simulink model "ScriptDemo"  (R2022b)
settings: configuration reference "TmVcThermal_Configuration_sub" (kept outside this file)
undefined symbols (not defined in the file or in its folder): aaaa, bbbb, cTmComprCtrl_D_u8HvacFlowTable_db, cTmComprCtrl_D_u8HvacFlowTable_sw, cTmComprCtrl_n_i16ChillCmpIMax, cTmComprCtrl_n_i16ChillCmpIMin, cTmComprCtrl_n_i16ChillCmpIMin666, cTmComprCtrl_n_i16ChillCmpPMax, cTmComprCtrl_n_i16ChillCmpPMin, cTmComprCtrl_n_i16CmpChillCoolRpmKiMax, cTmComprCtrl_n_i16CmpChillCoolRpmKiMin, cTmComprCtrl_n_i16CmpChillCoolRpmKpMax, cTmComprCtrl_n_i16CmpChillCoolRpmKpMin, cTmComprCtrl_n_i16CmpCoolRpmKiMax, cTmComprCtrl_n_i16CmpCoolRpmKiMin, cTmComprCtrl_n_i16CmpCoolRpmKpMax, cTmComprCtrl_n_i16CmpCoolRpmKpMin, cTmComprCtrl_n_i16SM4CmpHeatKiMax, cTmComprCtrl_n_i16SM4CmpHeatKiMin, cTmComprCtrl_n_i16SM4CmpHeatKpMax, cTmComprCtrl_n_i16SM4CmpHeatKpMin, cTmComprCtrl_n_i16SM5CmpHeatKiMax, cTmComprCtrl_n_i16SM5CmpHeatKiMin, cTmComprCtrl_n_i16SM5CmpHeatKpMax, cTmComprCtrl_n_i16SM5CmpHeatKpMin, cTmComprCtrl_n_i16SM6CmpHeatKiMax, cTmComprCtrl_n_i16SM6CmpHeatKiMin, cTmComprCtrl_n_i16SM6CmpHeatKpMax, cTmComprCtrl_n_i16SM6CmpHeatKpMin, cTmComprCtrl_n_u16CmpMaxSpdFanFltLimt, cTmComprCtrl_n_u16CmpMaxSpdLoSidePFltLimt, cTmComprCtrl_n_u16CmpMaxSpdSensorFltLimt, cTmComprCtrl_n_u16CompMinRpm, cTmComprCtrl_n_u16CompRpmIncThres, cTmComprCtrl_t_u16BattCooltFFPeriod, cTmComprCtrl_t_u16BattCooltPIPeriod, cTmComprCtrl_t_u16CmpCoolFFPeriod, cTmComprCtrl_t_u16CmpCoolPIPeriod, cTmComprCtrl_t_u16CoolCmpChillFFPeriod, cTmComprCtrl_t_u16CoolCmpChillPIPeriod, cTmComprCtrl_t_u16SM4CmpHeatFFPeriod, cTmComprCtrl_t_u16SM4CmpHeatPIPeriod, cTmComprCtrl_t_u16SM5CmpHeatFFPeriod, cTmComprCtrl_t_u16SM5CmpHeatPIPeriod, cTmComprCtrl_t_u16SM6CmpHeatFFPeriod, cTmComprCtrl_t_u16SM6CmpHeatPIPeriod, cTmComprCtrl_Te_EvapClearInteg, cTmComprCtrl_Te_i16HpReqTempSaturoffset, cTmComprCtrl_Te_i16SatLpReplaceDiff, cTmComprCtrl_Te_i16SM3BatDiffStartEvapDecOffset, cTmComprCtrl_Te_i16SM3EvapLo, cTmComprCtrl_Te_i16SM3TBatDiffEntEvapDecOffset, cTmComprCtrl_Te_i16SM3TBatDiffEntEvapDecOffsetQuit, cTmComprCtrl_Te_s32ErrCmpChillPIContinueCoolH, cTmComprCtrl_Te_s32ErrCmpChillPIContinueCoolL, cTmComprCtrl_Te_s32ErrCmpPIContinueChillH, cTmComprCtrl_Te_s32ErrCmpPIContinueChillL, cTmComprCtrl_Te_s32ErrCmpPIContinueCoolH, cTmComprCtrl_Te_s32ErrCmpPIContinueCoolL, cTmComprCtrl_Te_s32ErrCmpPIContinueHeatH ... (+398)
libraries: simulink x846, PCMULib x711, simulink_need_slupdate x4
(part 1 of 49)
settings Model: PacingRate=56  Creator=blue.ge  LastModifiedBy=blue.ge
settings ConfigSetRef: SourceName=TmVcThermal_Configuration_sub  SourceLocation=Base Workspace

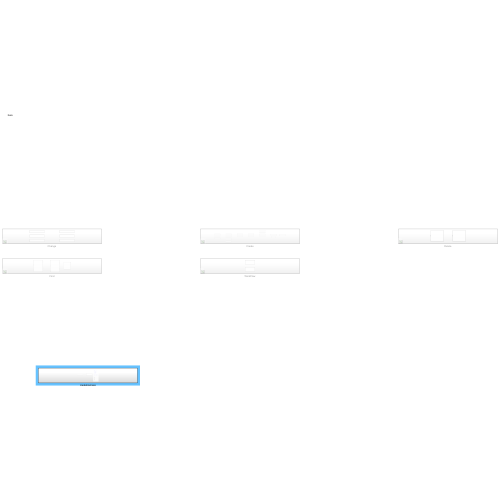
[thumbnail: Simulink's stored preview of the top-level diagram]
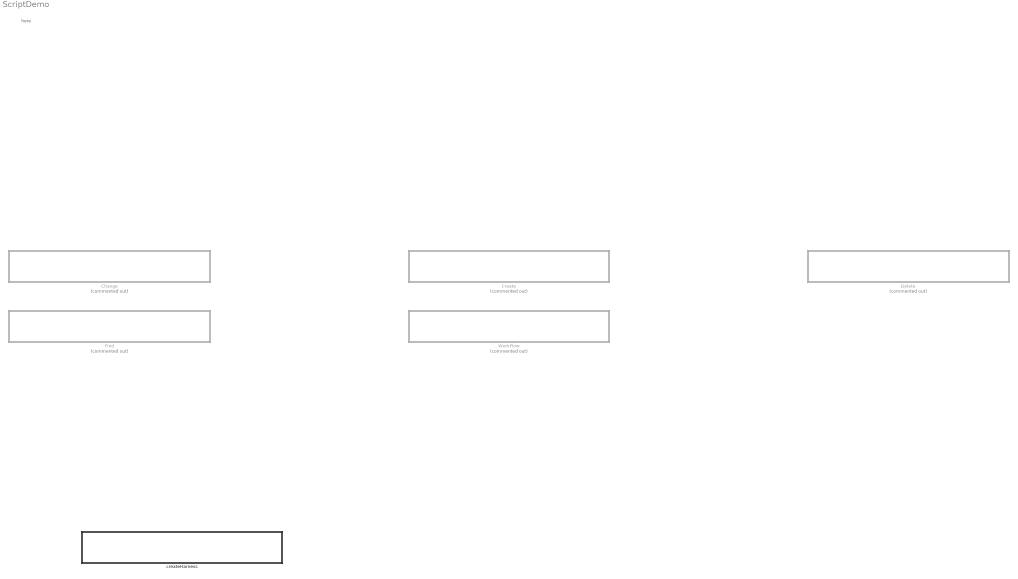
== system ScriptDemo ==
  note: here
  Change : Subsystem  Commented=on
  Create : Subsystem  Commented=on
  Delete : Subsystem  Commented=on
  Find : Subsystem  Commented=on
  WorkFlow : Subsystem  Commented=on
  createHarness : Subsystem

== system ScriptDemo/Change ==
  changeModPortName : Subsystem
  changeModPortType : Subsystem
  changeModSize : Subsystem
  changeModSizeGcs : Subsystem
  changePortBlockPosAll : Subsystem
  changeSigType : Subsystem

== system ScriptDemo/Create ==
  Model : Subsystem
  creatIFIn : Subsystem
  creatIFOut : Subsystem
  creatTmBase : Subsystem
  creatTmBaseArch : Subsystem
  creatTmIn : Subsystem
  creatTmOut : Subsystem
  createBus : Subsystem
  createDebug : Subsystem
  createGotoBasedPorts : Subsystem
  createGotoUseless : Subsystem
  createHarness : Subsystem
  createMerge : Subsystem
  createPorts : Subsystem
  createSigOnLine : Subsystem
  createStoreMem : Subsystem
  createSubMod : Subsystem
  createSubmodInfo : Subsystem
  createSwitchCase : Subsystem

== system ScriptDemo/Delete ==
  delUselessLine : Subsystem
  delUselessPort : Subsystem

== system ScriptDemo/Find ==
  findModBkConnected : Subsystem
  findModBkSpecific : Subsystem
  findNameMdOut : Subsystem

== system ScriptDemo/WorkFlow ==
  Step1_CreateSoftwareReq : Subsystem
  Step1_CreateSubModel : Subsystem

== system ScriptDemo/createHarness ==
  note: % 运行此脚本的时候，需要确保模型仿真通过, 可临时屏蔽其它案例或者将此模型复制到新的空白模型中
      |
      | createHarness(gcb, ...
      | 'lastStep' , 'Initialize' , ... % Initialize
      | 'mask' ,false, ...
      | 'lev1' ,{ 'NHP' , 'HP' }, ...
      | 'lev2' ,{ ...
      | { 'NoLimit' , 'Limit' }, ...
      | { 'NoLimit' , 'Limit' , 'Limit2' , 'Limit3' }, ...
      | }, ...
      | 'inName' ,{ ...
      | {
      | 'sTmIn_D_u8HeatPump' , ...
      | 'sTmDiag_D_u8HiSidePNHPFltSt' , ...
      | }, ...
      | {
      | 'sTmIn_D_u8HeatPump' , ...
      | 'sTmDiag_D_u8HiSidePFltSt' , ...
      | 'sTmDiag_D_u8OutrCondOutTFltSt' , ...
      | 'sTmDiag_D_u8CmprDischrgTFltSt' , ...
      | }, ...
      | }, ...
      | 'rstName' ,{ ...
      | {
      | 'rTmComprCtrl_n_u16CompMaxRpmSensFlt' ...
      | 'xTmComprCtrl_B_CmpSensorFltLimtFlag' ...
      | }, ...
      | {
      | 'rTmComprCtrl_n_u16CompMaxRpmSensFlt' ...
      | 'xTmComprCtrl_B_CmpSensorFltLimtFlag' ...
      | }, ...
      | }, ...
      | 'inValue' ,{ ...
      | { ...
      | {1 0 }, ...
      | {1 [1 2 3] }, ...
      | }, ...
      | { ...
      | {2 0 0 0 }, ...
      | {2 1 0 0 }, ...
      | {2 0 1 0 }, ...
      | {2 0 0 1 }, ...
      | }, ...
      | }, ...
      | 'rstValue' ,{ ...
      | { ...
      | {8000 false}, ...
      | {3000 true}, ...
      | }, ...
      | { ...
      | {8000 false}, ...
      | {3000 true}, ...
      | {3000 true}, ...
      | {3000 true}, ...
      | }, ...
      | } ...
      | )
  After : Subsystem
  Before : Subsystem  Commented=on
  Blue : Subsystem  Commented=on
  ID31659_OffCodeState : Subsystem

== system ScriptDemo/Change/changeModPortName ==
  After : Subsystem
  Before : Subsystem

== system ScriptDemo/Change/changeModPortType ==
  After : Subsystem
  Before : Subsystem

== system ScriptDemo/Change/changeModSize ==
  After : Subsystem
  Before : Subsystem

== system ScriptDemo/Change/changeModSizeGcs ==
  Before : Subsystem
  Before1 : Subsystem

== system ScriptDemo/Change/changePortBlockPosAll ==
  After1 : Subsystem
  Before : Subsystem

== system ScriptDemo/Change/changeSigType ==
  Before : Subsystem
  Before1 : Subsystem

== system ScriptDemo/Create/Model ==
  createModGoto : Subsystem
  createModGotoAll : Subsystem
  createModGroundTerm : Subsystem
  createModPorts : Subsystem
  createModSig : Subsystem
  createMode : Subsystem

== system ScriptDemo/Create/creatIFIn ==
  After : Subsystem
  Before : Subsystem

== system ScriptDemo/Create/creatIFOut ==
  After : Subsystem
  Before : Subsystem

== system ScriptDemo/Create/creatTmBase ==
  After : Subsystem
  Before : Subsystem

== system ScriptDemo/Create/creatTmBaseArch ==
  After : Subsystem
  Before : Subsystem

== system ScriptDemo/Create/creatTmIn ==
  After : Subsystem
  Before : Subsystem

== system ScriptDemo/Create/creatTmOut ==
  Before : Subsystem
  TmBase2Out : Subsystem
  wires:
  [sTmComprCtrl_n_u16CompRpmReq] -> TmBase2Out/1(sTmComprCtrl_n_u16CompRpmReq)
  [yTmComprCtrl_B_CompOnReq] -> TmBase2Out/2(yTmComprCtrl_B_CompOnReq)
  [sTmEnergyMgr_Pw_s32AcCmprPwrLim] -> TmBase2Out/3(sTmEnergyMgr_Pw_s32AcCmprPwrLim)
  [sTmRefriVlvCtrl_X_s32EEXVPosReq] -> TmBase2Out/4(sTmRefriVlvCtrl_X_s32EEXVPosReq)
  [yTmRefriVlvCtrl_B_EexvCalibReq] -> TmBase2Out/5(yTmRefriVlvCtrl_B_EexvCalibReq)
  [yTmRefriVlvCtrl_B_HpcEexvMovEnable] -> TmBase2Out/6(yTmRefriVlvCtrl_B_HpcEexvMovEnable)
  [sTmRefriVlvCtrl_X_s32BEXVPosReq] -> TmBase2Out/7(sTmRefriVlvCtrl_X_s32BEXVPosReq)
  [yTmRefriVlvCtrl_B_BexvCalibReq] -> TmBase2Out/8(yTmRefriVlvCtrl_B_BexvCalibReq)
  [yTmRefriVlvCtrl_B_HpcBexvMovEnable] -> TmBase2Out/9(yTmRefriVlvCtrl_B_HpcBexvMovEnable)
  [sTmRefriVlvCtrl_X_s32CEXVPosReq] -> TmBase2Out/10(sTmRefriVlvCtrl_X_s32CEXVPosReq)
  [yTmRefriVlvCtrl_B_CexvCalibReq] -> TmBase2Out/11(yTmRefriVlvCtrl_B_CexvCalibReq)
  [yTmRefriVlvCtrl_B_HpcCexvMovEnable] -> TmBase2Out/12(yTmRefriVlvCtrl_B_HpcCexvMovEnable)
  [sTmColtVlvCtrl_D_u8HpcBctvRefDrvReq] -> TmBase2Out/13(sTmColtVlvCtrl_D_u8HpcBctvRefDrvReq)
  [sTmColtVlvCtrl_X_u8BctvPosReq] -> TmBase2Out/14(sTmColtVlvCtrl_X_u8BctvPosReq)
  [sTmColtVlvCtrl_D_u8HpcBcfvRefDrvReq] -> TmBase2Out/15(sTmColtVlvCtrl_D_u8HpcBcfvRefDrvReq)
  [sTmDiag_D_u8VcEvLowSidePSnrSB] -> TmBase2Out/16(sTmDiag_D_u8VcEvLowSidePSnrSB)
  [sTmDiag_D_u8VcEvLowSidePSnrOP] -> TmBase2Out/17(sTmDiag_D_u8VcEvLowSidePSnrOP)
  [sTmDiag_D_u8VcEvHiSidePSnrOP] -> TmBase2Out/18(sTmDiag_D_u8VcEvHiSidePSnrOP)
  [sTmDiag_D_u8VcEvHiSidePSnrSB] -> TmBase2Out/19(sTmDiag_D_u8VcEvHiSidePSnrSB)
  [sTmDiag_D_u8VcEvHiSideTmpSnrSG] -> TmBase2Out/20(sTmDiag_D_u8VcEvHiSideTmpSnrSG)
  [sTmDiag_D_u8VcEvHiSideTmpSnrOP] -> TmBase2Out/21(sTmDiag_D_u8VcEvHiSideTmpSnrOP)
  [sTmDiag_D_u8VcEvBattCooltLvlLo] -> TmBase2Out/22(sTmDiag_D_u8VcEvBattCooltLvlLo)
  [sTmDiag_D_u8VcEvSov1SB] -> TmBase2Out/23(sTmDiag_D_u8VcEvSov1SB)
  [sTmDiag_D_u8VcEvSov2SB] -> TmBase2Out/24(sTmDiag_D_u8VcEvSov2SB)
  [sTmDiag_D_u8VcEvSov3SB] -> TmBase2Out/25(sTmDiag_D_u8VcEvSov3SB)
  [sTmDiag_D_u8VcEvSov5SB] -> TmBase2Out/26(sTmDiag_D_u8VcEvSov5SB)
  [sTmDiag_D_u8VcEvSov4SB] -> TmBase2Out/27(sTmDiag_D_u8VcEvSov4SB)
  [sTmDiag_D_u8VcEvSBFan] -> TmBase2Out/28(sTmDiag_D_u8VcEvSBFan)
  [sTmDiag_D_u8VcEvOPFan] -> TmBase2Out/29(sTmDiag_D_u8VcEvOPFan)
  [sTmDiag_D_u8VcEvSGFan] -> TmBase2Out/30(sTmDiag_D_u8VcEvSGFan)
  [sTmDiag_D_u8VcEvVolErrFan] -> TmBase2Out/31(sTmDiag_D_u8VcEvVolErrFan)
  [sTmDiag_D_u8VcEvBlokFan] -> TmBase2Out/32(sTmDiag_D_u8VcEvBlokFan)
  [sTmDiag_D_u8VcEvCircutInteFlt] -> TmBase2Out/33(sTmDiag_D_u8VcEvCircutInteFlt)
  [sTmDiag_D_u8VcEvHmPumpSB] -> TmBase2Out/34(sTmDiag_D_u8VcEvHmPumpSB)
  [sTmDiag_D_u8VcEvHmPumpOC] -> TmBase2Out/35(sTmDiag_D_u8VcEvHmPumpOC)
  [sTmDiag_D_u8HpmSov1Actv2FEnState] -> TmBase2Out/36(sTmDiag_D_u8HpmSov1Actv2FEnState)
  [sTmDiag_D_u8HpmSov2Actv2FEnState] -> TmBase2Out/37(sTmDiag_D_u8HpmSov2Actv2FEnState)
  [sTmDiag_D_u8HpmSov3Actv2FEnState] -> TmBase2Out/38(sTmDiag_D_u8HpmSov3Actv2FEnState)
  [sTmDiag_D_u8FanPwm2FEnState] -> TmBase2Out/39(sTmDiag_D_u8FanPwm2FEnState)
  [sTmDiag_D_u8BattCooltPmp2FEnState] -> TmBase2Out/40(sTmDiag_D_u8BattCooltPmp2FEnState)
  [sTmDiag_D_u8EmCooltPmp2FEnState] -> TmBase2Out/41(sTmDiag_D_u8EmCooltPmp2FEnState)
  [sTmDiag_D_u8PTCPumpSpd2FEnState] -> TmBase2Out/42(sTmDiag_D_u8PTCPumpSpd2FEnState)
  [sTmDiag_D_u8EctvVlvMoveEna2FEnaState] -> TmBase2Out/43(sTmDiag_D_u8EctvVlvMoveEna2FEnaState)
  [sTmDiag_D_u8EctvVlvPos2FEnaState] -> TmBase2Out/44(sTmDiag_D_u8EctvVlvPos2FEnaState)
  [sTmDiag_D_u8BctvVlvRef2FEnaState] -> TmBase2Out/45(sTmDiag_D_u8BctvVlvRef2FEnaState)
  [sTmDiag_D_u8BctvVlvPos2FEnaState] -> TmBase2Out/46(sTmDiag_D_u8BctvVlvPos2FEnaState)
  [sTmDiag_D_u8BcfvVlvRef2FEnaState] -> TmBase2Out/47(sTmDiag_D_u8BcfvVlvRef2FEnaState)
  [sTmDiag_D_u8BcfvVlvPos2FEnaState] -> TmBase2Out/48(sTmDiag_D_u8BcfvVlvPos2FEnaState)
  [sTmDiag_D_u8BexvCal2FEnaState] -> TmBase2Out/49(sTmDiag_D_u8BexvCal2FEnaState)
  [sTmDiag_D_u8BexvMoveEna2FEnaState] -> TmBase2Out/50(sTmDiag_D_u8BexvMoveEna2FEnaState)
  [sTmDiag_D_u8BexvPosnReq2FEnaState] -> TmBase2Out/51(sTmDiag_D_u8BexvPosnReq2FEnaState)
  [sTmDiag_D_u8CexvCal2FEnaState] -> TmBase2Out/52(sTmDiag_D_u8CexvCal2FEnaState)
  [sTmDiag_D_u8CexvMoveEna2FEnaState] -> TmBase2Out/53(sTmDiag_D_u8CexvMoveEna2FEnaState)
  [sTmDiag_D_u8CexvPosnReq2FEnaState] -> TmBase2Out/54(sTmDiag_D_u8CexvPosnReq2FEnaState)
  [sTmDiag_D_u8EexvCal2FEnaState] -> TmBase2Out/55(sTmDiag_D_u8EexvCal2FEnaState)
  TmBase2Out/1(sTmOut_n_u16ElacCmprReq) -> [sTmOut_n_u16ElacCmprReq]
  TmBase2Out/2(sTmOut_D_u8ElacCmprRelease) -> [sTmOut_D_u8ElacCmprRelease]
  TmBase2Out/3(sTmOut_Pw_s32ElacCmprMax) -> [sTmOut_Pw_s32ElacCmprMax]
  TmBase2Out/4(sTmOut_X_s32EexvVlvPosReq) -> [sTmOut_X_s32EexvVlvPosReq]
  TmBase2Out/5(yTmOut_B_EexvPosnCalibReq) -> [yTmOut_B_EexvPosnCalibReq]
  TmBase2Out/6(yTmOut_B_EexvPosnMovEnable) -> [yTmOut_B_EexvPosnMovEnable]
  TmBase2Out/7(sTmOut_X_s32BexvVlvPosReq) -> [sTmOut_X_s32BexvVlvPosReq]
  TmBase2Out/8(yTmOut_B_BexvPosnCalibReq) -> [yTmOut_B_BexvPosnCalibReq]
  TmBase2Out/9(yTmOut_B_BexvPosnMovEnable) -> [yTmOut_B_BexvPosnMovEnable]
  TmBase2Out/10(sTmOut_X_s32CexvVlvPosReq) -> [sTmOut_X_s32CexvVlvPosReq]
  TmBase2Out/11(yTmOut_B_CexvPosnCalibReq) -> [yTmOut_B_CexvPosnCalibReq]
  TmBase2Out/12(yTmOut_B_CexvPosnMovEnable) -> [yTmOut_B_CexvPosnMovEnable]
  TmBase2Out/13(sTmOut_D_u8BctvVlvRefDrvReq) -> [sTmOut_D_u8BctvVlvRefDrvReq]
  TmBase2Out/14(sTmOut_X_u8BctvVlvPosReq) -> [sTmOut_X_u8BctvVlvPosReq]
  TmBase2Out/15(sTmOut_D_u8BcfvVlvRefDrvReq) -> [sTmOut_D_u8BcfvVlvRefDrvReq]
  TmBase2Out/16(sTmOut_D_u8VcEvLowSidePSnrSB) -> [sTmOut_D_u8VcEvLowSidePSnrSB]
  TmBase2Out/17(sTmOut_D_u8VcEvLowSidePSnrOP) -> [sTmOut_D_u8VcEvLowSidePSnrOP]
  TmBase2Out/18(sTmOut_D_u8VcEvHiSidePSnrOP) -> [sTmOut_D_u8VcEvHiSidePSnrOP]
  TmBase2Out/19(sTmOut_D_u8VcEvHiSidePSnrSB) -> [sTmOut_D_u8VcEvHiSidePSnrSB]
  TmBase2Out/20(sTmOut_D_u8VcEvHiSideTmpSnrSG) -> [sTmOut_D_u8VcEvHiSideTmpSnrSG]
  TmBase2Out/21(sTmOut_D_u8VcEvHiSideTmpSnrOP) -> [sTmOut_D_u8VcEvHiSideTmpSnrOP]
  TmBase2Out/22(sTmOut_D_u8VcEvBattCooltLvlLo) -> [sTmOut_D_u8VcEvBattCooltLvlLo]
  TmBase2Out/23(sTmOut_D_u8VcEvSov1SB) -> [sTmOut_D_u8VcEvSov1SB]
  TmBase2Out/24(sTmOut_D_u8VcEvSov2SB) -> [sTmOut_D_u8VcEvSov2SB]
  TmBase2Out/25(sTmOut_D_u8VcEvSov3SB) -> [sTmOut_D_u8VcEvSov3SB]
  TmBase2Out/26(sTmOut_D_u8VcEvSov5SB) -> [sTmOut_D_u8VcEvSov5SB]
  TmBase2Out/27(sTmOut_D_u8VcEvSov4SB) -> [sTmOut_D_u8VcEvSov4SB]
  TmBase2Out/28(sTmOut_D_u8VcEvSBFan) -> [sTmOut_D_u8VcEvSBFan]
  TmBase2Out/29(sTmOut_D_u8VcEvOPFan) -> [sTmOut_D_u8VcEvOPFan]
  TmBase2Out/30(sTmOut_D_u8VcEvSGFan) -> [sTmOut_D_u8VcEvSGFan]
  TmBase2Out/31(sTmOut_D_u8VcEvVolErrFan) -> [sTmOut_D_u8VcEvVolErrFan]
  TmBase2Out/32(sTmOut_D_u8VcEvBlokFan) -> [sTmOut_D_u8VcEvBlokFan]
  TmBase2Out/33(sTmOut_D_u8VcEvCircutInteFlt) -> [sTmOut_D_u8VcEvCircutInteFlt]
  TmBase2Out/34(sTmOut_D_u8VcEvHmPumpSB) -> [sTmOut_D_u8VcEvHmPumpSB]
  TmBase2Out/35(sTmOut_D_u8VcEvHmPumpOC) -> [sTmOut_D_u8VcEvHmPumpOC]
  TmBase2Out/36(sTmOut_D_u8HpmSov1Actv2FEnState) -> [sTmOut_D_u8HpmSov1Actv2FEnState]
  TmBase2Out/37(sTmOut_D_u8HpmSov2Actv2FEnState) -> [sTmOut_D_u8HpmSov2Actv2FEnState]
  TmBase2Out/38(sTmOut_D_u8HpmSov3Actv2FEnState) -> [sTmOut_D_u8HpmSov3Actv2FEnState]
  TmBase2Out/39(sTmOut_D_u8FanPwm2FEnState) -> [sTmOut_D_u8FanPwm2FEnState]
  TmBase2Out/40(sTmOut_D_u8BattCooltPmp2FEnState) -> [sTmOut_D_u8BattCooltPmp2FEnState]
  TmBase2Out/41(sTmOut_D_u8EmCooltPmp2FEnState) -> [sTmOut_D_u8EmCooltPmp2FEnState]
  TmBase2Out/42(sTmOut_D_u8PTCPumpSpd2FEnState) -> [sTmOut_D_u8PTCPumpSpd2FEnState]
  TmBase2Out/43(sTmOut_D_u8EctvVlvMoveEna2FEnaState) -> [sTmOut_D_u8EctvVlvMoveEna2FEnaState]
  TmBase2Out/44(sTmOut_D_u8EctvVlvPos2FEnaState) -> [sTmOut_D_u8EctvVlvPos2FEnaState]
  TmBase2Out/45(sTmOut_D_u8BctvVlvRef2FEnaState) -> [sTmOut_D_u8BctvVlvRef2FEnaState]
  TmBase2Out/46(sTmOut_D_u8BctvVlvPos2FEnaState) -> [sTmOut_D_u8BctvVlvPos2FEnaState]
  TmBase2Out/47(sTmOut_D_u8BcfvVlvRef2FEnaState) -> [sTmOut_D_u8BcfvVlvRef2FEnaState]
  TmBase2Out/48(sTmOut_D_u8BcfvVlvPos2FEnaState) -> [sTmOut_D_u8BcfvVlvPos2FEnaState]
  TmBase2Out/49(sTmOut_D_u8BexvCal2FEnaState) -> [sTmOut_D_u8BexvCal2FEnaState]
  TmBase2Out/50(sTmOut_D_u8BexvMoveEna2FEnaState) -> [sTmOut_D_u8BexvMoveEna2FEnaState]
  TmBase2Out/51(sTmOut_D_u8BexvPosnReq2FEnaState) -> [sTmOut_D_u8BexvPosnReq2FEnaState]
  TmBase2Out/52(sTmOut_D_u8CexvCal2FEnaState) -> [sTmOut_D_u8CexvCal2FEnaState]
  TmBase2Out/53(sTmOut_D_u8CexvMoveEna2FEnaState) -> [sTmOut_D_u8CexvMoveEna2FEnaState]
  TmBase2Out/54(sTmOut_D_u8CexvPosnReq2FEnaState) -> [sTmOut_D_u8CexvPosnReq2FEnaState]
  TmBase2Out/55(sTmOut_D_u8EexvCal2FEnaState) -> [sTmOut_D_u8EexvCal2FEnaState]

== system ScriptDemo/Create/createBus ==
  createBusGoto : Subsystem
  createBusPort : Subsystem

== system ScriptDemo/Create/createDebug ==
  After : Subsystem
  After1 : Subsystem
  Before : Subsystem
  Before1 : Subsystem

== system ScriptDemo/Create/createGotoBasedPorts ==
  After : Subsystem
  Before : Subsystem

== system ScriptDemo/Create/createGotoUseless ==
  After : Subsystem
  Before : Subsystem

== system ScriptDemo/Create/createHarness ==
  note: % 运行此脚本的时候，需要确保模型仿真通过, 可临时屏蔽其它案例或者将此模型复制到新的空白模型中
      |
      | createHarness(gcb, ...
      | 'lastStep' , 'Initialize' , ... % Initialize
      | 'mask' ,false, ...
      | 'lev1' ,{ 'NHP' , 'HP' }, ...
      | 'lev2' ,{ ...
      | { 'NoLimit' , 'Limit' }, ...
      | { 'NoLimit' , 'Limit' , 'Limit2' , 'Limit3' }, ...
      | }, ...
      | 'inName' ,{ ...
      | {
      | 'sTmIn_D_u8HeatPump' , ...
      | 'sTmDiag_D_u8HiSidePNHPFltSt' , ...
      | }, ...
      | {
      | 'sTmIn_D_u8HeatPump' , ...
      | 'sTmDiag_D_u8HiSidePFltSt' , ...
      | 'sTmDiag_D_u8OutrCondOutTFltSt' , ...
      | 'sTmDiag_D_u8CmprDischrgTFltSt' , ...
      | }, ...
      | }, ...
      | 'rstName' ,{ ...
      | {
      | 'rTmComprCtrl_n_u16CompMaxRpmSensFlt' ...
      | 'xTmComprCtrl_B_CmpSensorFltLimtFlag' ...
      | }, ...
      | {
      | 'rTmComprCtrl_n_u16CompMaxRpmSensFlt' ...
      | 'xTmComprCtrl_B_CmpSensorFltLimtFlag' ...
      | }, ...
      | }, ...
      | 'inValue' ,{ ...
      | { ...
      | {1 0 }, ...
      | {1 [1 2 3] }, ...
      | }, ...
      | { ...
      | {2 0 0 0 }, ...
      | {2 1 0 0 }, ...
      | {2 0 1 0 }, ...
      | {2 0 0 1 }, ...
      | }, ...
      | }, ...
      | 'rstValue' ,{ ...
      | { ...
      | {8000 false}, ...
      | {3000 true}, ...
      | }, ...
      | { ...
      | {8000 false}, ...
      | {3000 true}, ...
      | {3000 true}, ...
      | {3000 true}, ...
      | }, ...
      | } ...
      | )
  After : Subsystem
  Before : Subsystem  Commented=on
  Blue : Subsystem  Commented=on
  ID31659_OffCodeState : Subsystem

== system ScriptDemo/Create/createMerge ==
  After : Subsystem
  Before : Subsystem

== system ScriptDemo/Create/createPorts ==
  createPorts : Subsystem
  createPortsGoto : Subsystem
  createPortsGotoUpdate : Subsystem
  createPortsGotoUpdateLoop : Subsystem

== system ScriptDemo/Create/createSigOnLine ==
  note: % 目的: 对模型输入输出端口的信号线进行解析
      | createSigOnLine (gcb, ...
      | 'isEnableIn' ,true, ...
      | 'isEnableOut' ,true, ...
      | 'resoveValue' ,false, ...
      | 'logValue' ,false, ...
      | 'testValue' ,false ...
      | )
  After : Subsystem
  After2 : Subsystem
  After3 : Subsystem
  After4 : Subsystem
  Before : Subsystem
  Before1 : Subsystem
  Before2 : Subsystem
  Before3 : Subsystem
  Before4 : Subsystem

== system ScriptDemo/Create/createStoreMem ==
  After : Subsystem

== system ScriptDemo/Create/createSubMod ==
  After : Subsystem

== system ScriptDemo/Create/createSubmodInfo ==
  After : Subsystem
  Before : Subsystem

== system ScriptDemo/Create/createSwitchCase ==
  After : Subsystem

== system ScriptDemo/Delete/delUselessLine ==
  In1 : Inport
  After : Subsystem
  Before : Subsystem

== system ScriptDemo/Delete/delUselessPort ==
  In1 : Inport
  After : Subsystem
  After1 : Subsystem
  Before : Subsystem

== system ScriptDemo/Find/findModBkConnected ==
  note: createSigOnLine(gcs ,'resoveValue',true)
  sTmRefriVlvCtrl_X_s32EEXVPosReqIn : Inport  OutDataTypeStr=single
  sTmRefriVlvCtrl_X_s32BEXVPosReqIn : Inport  Port=2  OutDataTypeStr=single
  yTmRefriVlvCtrl_B_HpcCexvMovEnableIn : Inport  Port=3  OutDataTypeStr=boolean
  sTmRefriVlvCtrl_Z_u8CEXVInitStateIn : Inport  Port=4  OutDataTypeStr=uint8
  yTmRefriVlvCtrl_B_CexvCalibReqIn : Inport  Port=5  OutDataTypeStr=boolean
  yTmRefriVlvCtrl_B_HpcEexvMovEnableIn : Inport  Port=6  OutDataTypeStr=boolean
  sTmRefriVlvCtrl_Z_u8EEXVInitStateIn : Inport  Port=7  OutDataTypeStr=uint8
  sTmRefriVlvCtrl_Z_u8BEXVInitStateIn : Inport  Port=8  OutDataTypeStr=uint8
  yTmRefriVlvCtrl_B_BexvCalibReqIn : Inport  Port=9  OutDataTypeStr=boolean
  sTmRefriVlvCtrl_X_s32SM3BexvMaxPosIn : Inport  Port=10  OutDataTypeStr=single
  yTmRefriVlvCtrl_B_EvapBattTLimBexvEnaIn : Inport  Port=11  OutDataTypeStr=boolean
  sTmRefriVlvCtrl_D_u8EexvRefriSwitchStIn : Inport  Port=12  OutDataTypeStr=uint8
  sTmRefriVlvCtrl_D_u8CexvRefriSwitchStIn : Inport  Port=13  OutDataTypeStr=uint8
  sTmRefriVlvCtrl_D_u8BexvRefriSwitchStIn : Inport  Port=14  OutDataTypeStr=uint8
  Before : Subsystem
  Ground : Ground
  Ground1 : Ground
  Terminator : Terminator
  Terminator1 : Terminator
  sTmRefriVlvCtrl_X_s32CEXVPosReq : Outport  OutDataTypeStr=single
  sTmRefriVlvCtrl_X_s32EEXVPosReq : Outport  Port=2  OutDataTypeStr=single
  sTmRefriVlvCtrl_X_s32BEXVPosReq : Outport  Port=3  OutDataTypeStr=single
  yTmRefriVlvCtrl_B_HpcCexvMovEnable : Outport  Port=4  OutDataTypeStr=boolean
  sTmRefriVlvCtrl_Z_u8CEXVInitState : Outport  Port=5  OutDataTypeStr=uint8
  yTmRefriVlvCtrl_B_CexvCalibReq : Outport  Port=6  OutDataTypeStr=boolean
  yTmRefriVlvCtrl_B_HpcEexvMovEnable : Outport  Port=7  OutDataTypeStr=boolean
  sTmRefriVlvCtrl_Z_u8EEXVInitState : Outport  Port=8  OutDataTypeStr=uint8
  sTmRefriVlvCtrl_Z_u8BEXVInitState : Outport  Port=9  OutDataTypeStr=uint8
  yTmRefriVlvCtrl_B_BexvCalibReq : Outport  Port=10  OutDataTypeStr=boolean
  sTmRefriVlvCtrl_X_s32SM3BexvMaxPos : Outport  Port=11  OutDataTypeStr=single
  yTmRefriVlvCtrl_B_EvapBattTLimBexvEna : Outport  Port=12  OutDataTypeStr=boolean
  sTmRefriVlvCtrl_D_u8EexvRefriSwitchSt : Outport  Port=13  OutDataTypeStr=uint8
  wires:
  Before/17(sTmRefriVlvCtrl_D_u8BexvRefriSwitchSt) -> Terminator1/1  "sTmRefriVlvCtrl_D_u8BexvRefriSwitchSt"
  Before/3(sTmRefriVlvCtrl_X_s32BEXVPosReq) -> sTmRefriVlvCtrl_X_s32BEXVPosReq/1  "sTmRefriVlvCtrl_X_s32BEXVPosReq"
  Before/11(sTmRefriVlvCtrl_Z_u8BEXVInitState) -> sTmRefriVlvCtrl_Z_u8BEXVInitState/1  "sTmRefriVlvCtrl_Z_u8BEXVInitState"
  Before/15(sTmRefriVlvCtrl_D_u8EexvRefriSwitchSt) -> sTmRefriVlvCtrl_D_u8EexvRefriSwitchSt/1  "sTmRefriVlvCtrl_D_u8EexvRefriSwitchSt"
  Before/7(yTmRefriVlvCtrl_B_HpcEexvMovEnable) -> yTmRefriVlvCtrl_B_HpcEexvMovEnable/1  "yTmRefriVlvCtrl_B_HpcEexvMovEnable"
  Before/14(yTmRefriVlvCtrl_B_EvapBattTLimBexvEna) -> yTmRefriVlvCtrl_B_EvapBattTLimBexvEna/1  "yTmRefriVlvCtrl_B_EvapBattTLimBexvEna"
  Before/12(yTmRefriVlvCtrl_B_BexvCalibReq) -> yTmRefriVlvCtrl_B_BexvCalibReq/1  "yTmRefriVlvCtrl_B_BexvCalibReq"
  Before/5(sTmRefriVlvCtrl_Z_u8CEXVInitState) -> sTmRefriVlvCtrl_Z_u8CEXVInitState/1  "sTmRefriVlvCtrl_Z_u8CEXVInitState"
  Before/13(sTmRefriVlvCtrl_X_s32SM3BexvMaxPos) -> sTmRefriVlvCtrl_X_s32SM3BexvMaxPos/1  "sTmRefriVlvCtrl_X_s32SM3BexvMaxPos"
  Before/4(yTmRefriVlvCtrl_B_HpcCexvMovEnable) -> yTmRefriVlvCtrl_B_HpcCexvMovEnable/1  "yTmRefriVlvCtrl_B_HpcCexvMovEnable"
  sTmRefriVlvCtrl_D_u8EexvRefriSwitchStIn/1 -> Before/15(sTmRefriVlvCtrl_D_u8EexvRefriSwitchStIn)  "sTmRefriVlvCtrl_D_u8EexvRefriSwitchStIn"
  yTmRefriVlvCtrl_B_CexvCalibReqIn/1 -> Before/6(yTmRefriVlvCtrl_B_CexvCalibReqIn)  "yTmRefriVlvCtrl_B_CexvCalibReqIn"
  sTmRefriVlvCtrl_D_u8BexvRefriSwitchStIn/1 -> Before/17(sTmRefriVlvCtrl_D_u8BexvRefriSwitchStIn)  "sTmRefriVlvCtrl_D_u8BexvRefriSwitchStIn"
  Before/16(sTmRefriVlvCtrl_D_u8CexvRefriSwitchSt) -> Terminator/1  "sTmRefriVlvCtrl_D_u8CexvRefriSwitchSt"
  Before/2(sTmRefriVlvCtrl_X_s32EEXVPosReq) -> sTmRefriVlvCtrl_X_s32EEXVPosReq/1  "sTmRefriVlvCtrl_X_s32EEXVPosReq"
  sTmRefriVlvCtrl_D_u8CexvRefriSwitchStIn/1 -> Before/16(sTmRefriVlvCtrl_D_u8CexvRefriSwitchStIn)  "sTmRefriVlvCtrl_D_u8CexvRefriSwitchStIn"
  yTmRefriVlvCtrl_B_HpcCexvMovEnableIn/1 -> Before/4(yTmRefriVlvCtrl_B_HpcCexvMovEnableIn)  "yTmRefriVlvCtrl_B_HpcCexvMovEnableIn"
  yTmRefriVlvCtrl_B_BexvCalibReqIn/1 -> Before/12(yTmRefriVlvCtrl_B_BexvCalibReqIn)  "yTmRefriVlvCtrl_B_BexvCalibReqIn"
  Before/6(yTmRefriVlvCtrl_B_CexvCalibReq) -> yTmRefriVlvCtrl_B_CexvCalibReq/1  "yTmRefriVlvCtrl_B_CexvCalibReq"
  sTmRefriVlvCtrl_X_s32SM3BexvMaxPosIn/1 -> Before/13(sTmRefriVlvCtrl_X_s32SM3BexvMaxPosIn)  "sTmRefriVlvCtrl_X_s32SM3BexvMaxPosIn"
  yTmRefriVlvCtrl_B_HpcEexvMovEnableIn/1 -> Before/7(yTmRefriVlvCtrl_B_HpcEexvMovEnableIn)  "yTmRefriVlvCtrl_B_HpcEexvMovEnableIn"
  Ground/1 -> Before/9(yTmRefriVlvCtrl_B_EexvCalibReqIn)  "yTmRefriVlvCtrl_B_EexvCalibReqIn"
  sTmRefriVlvCtrl_Z_u8CEXVInitStateIn/1 -> Before/5(sTmRefriVlvCtrl_Z_u8CEXVInitStateIn)  "sTmRefriVlvCtrl_Z_u8CEXVInitStateIn"
  sTmRefriVlvCtrl_Z_u8BEXVInitStateIn/1 -> Before/11(sTmRefriVlvCtrl_Z_u8BEXVInitStateIn)  "sTmRefriVlvCtrl_Z_u8BEXVInitStateIn"
  sTmRefriVlvCtrl_X_s32BEXVPosReqIn/1 -> Before/3(sTmRefriVlvCtrl_X_s32BEXVPosReqIn)  "sTmRefriVlvCtrl_X_s32BEXVPosReqIn"
  Before/1(sTmRefriVlvCtrl_X_s32CEXVPosReq) -> sTmRefriVlvCtrl_X_s32CEXVPosReq/1  "sTmRefriVlvCtrl_X_s32CEXVPosReq"
  Ground1/1 -> Before/10(yTmRefriVlvCtrl_B_HpcBexvMovEnableIn)  "yTmRefriVlvCtrl_B_HpcBexvMovEnableIn"
  sTmRefriVlvCtrl_X_s32EEXVPosReqIn/1 -> Before/2(sTmRefriVlvCtrl_X_s32EEXVPosReqIn)  "sTmRefriVlvCtrl_X_s32EEXVPosReqIn"
  sTmRefriVlvCtrl_Z_u8EEXVInitStateIn/1 -> Before/8(sTmRefriVlvCtrl_Z_u8EEXVInitStateIn)  "sTmRefriVlvCtrl_Z_u8EEXVInitStateIn"
  Before/8(sTmRefriVlvCtrl_Z_u8EEXVInitState) -> sTmRefriVlvCtrl_Z_u8EEXVInitState/1  "sTmRefriVlvCtrl_Z_u8EEXVInitState"
  yTmRefriVlvCtrl_B_EvapBattTLimBexvEnaIn/1 -> Before/14(yTmRefriVlvCtrl_B_EvapBattTLimBexvEnaIn)  "yTmRefriVlvCtrl_B_EvapBattTLimBexvEnaIn"

== system ScriptDemo/Find/findModBkSpecific ==
  note: createSigOnLine(gcs ,'resoveValue',true)
  sTmRefriVlvCtrl_X_s32EEXVPosReqIn : Inport  OutDataTypeStr=single
  sTmRefriVlvCtrl_X_s32BEXVPosReqIn : Inport  Port=2  OutDataTypeStr=single
  yTmRefriVlvCtrl_B_HpcCexvMovEnableIn : Inport  Port=3  OutDataTypeStr=boolean
  sTmRefriVlvCtrl_Z_u8CEXVInitStateIn : Inport  Port=4  OutDataTypeStr=uint8
  yTmRefriVlvCtrl_B_CexvCalibReqIn : Inport  Port=5  OutDataTypeStr=boolean
  yTmRefriVlvCtrl_B_HpcEexvMovEnableIn : Inport  Port=6  OutDataTypeStr=boolean
  sTmRefriVlvCtrl_Z_u8EEXVInitStateIn : Inport  Port=7  OutDataTypeStr=uint8
  sTmRefriVlvCtrl_Z_u8BEXVInitStateIn : Inport  Port=8  OutDataTypeStr=uint8
  yTmRefriVlvCtrl_B_BexvCalibReqIn : Inport  Port=9  OutDataTypeStr=boolean
  sTmRefriVlvCtrl_X_s32SM3BexvMaxPosIn : Inport  Port=10  OutDataTypeStr=single
  yTmRefriVlvCtrl_B_EvapBattTLimBexvEnaIn : Inport  Port=11  OutDataTypeStr=boolean
  sTmRefriVlvCtrl_D_u8EexvRefriSwitchStIn : Inport  Port=12  OutDataTypeStr=uint8
  sTmRefriVlvCtrl_D_u8CexvRefriSwitchStIn : Inport  Port=13  OutDataTypeStr=uint8
  sTmRefriVlvCtrl_D_u8BexvRefriSwitchStIn : Inport  Port=14  OutDataTypeStr=uint8
  Before : Subsystem
  Ground : Ground
  Ground1 : Ground
  Terminator : Terminator
  Terminator1 : Terminator
  sTmRefriVlvCtrl_X_s32CEXVPosReq : Outport  OutDataTypeStr=single
  sTmRefriVlvCtrl_X_s32EEXVPosReq : Outport  Port=2  OutDataTypeStr=single
  sTmRefriVlvCtrl_X_s32BEXVPosReq : Outport  Port=3  OutDataTypeStr=single
  yTmRefriVlvCtrl_B_HpcCexvMovEnable : Outport  Port=4  OutDataTypeStr=boolean
  sTmRefriVlvCtrl_Z_u8CEXVInitState : Outport  Port=5  OutDataTypeStr=uint8
  yTmRefriVlvCtrl_B_CexvCalibReq : Outport  Port=6  OutDataTypeStr=boolean
  yTmRefriVlvCtrl_B_HpcEexvMovEnable : Outport  Port=7  OutDataTypeStr=boolean
  sTmRefriVlvCtrl_Z_u8EEXVInitState : Outport  Port=8  OutDataTypeStr=uint8
  sTmRefriVlvCtrl_Z_u8BEXVInitState : Outport  Port=9  OutDataTypeStr=uint8
  yTmRefriVlvCtrl_B_BexvCalibReq : Outport  Port=10  OutDataTypeStr=boolean
  sTmRefriVlvCtrl_X_s32SM3BexvMaxPos : Outport  Port=11  OutDataTypeStr=single
  yTmRefriVlvCtrl_B_EvapBattTLimBexvEna : Outport  Port=12  OutDataTypeStr=boolean
  sTmRefriVlvCtrl_D_u8EexvRefriSwitchSt : Outport  Port=13  OutDataTypeStr=uint8
  wires:
  Before/17(sTmRefriVlvCtrl_D_u8BexvRefriSwitchSt) -> Terminator1/1  "sTmRefriVlvCtrl_D_u8BexvRefriSwitchSt"
  Before/3(sTmRefriVlvCtrl_X_s32BEXVPosReq) -> sTmRefriVlvCtrl_X_s32BEXVPosReq/1  "sTmRefriVlvCtrl_X_s32BEXVPosReq"
  Before/11(sTmRefriVlvCtrl_Z_u8BEXVInitState) -> sTmRefriVlvCtrl_Z_u8BEXVInitState/1  "sTmRefriVlvCtrl_Z_u8BEXVInitState"
  Before/15(sTmRefriVlvCtrl_D_u8EexvRefriSwitchSt) -> sTmRefriVlvCtrl_D_u8EexvRefriSwitchSt/1  "sTmRefriVlvCtrl_D_u8EexvRefriSwitchSt"
  Before/7(yTmRefriVlvCtrl_B_HpcEexvMovEnable) -> yTmRefriVlvCtrl_B_HpcEexvMovEnable/1  "yTmRefriVlvCtrl_B_HpcEexvMovEnable"
  Before/14(yTmRefriVlvCtrl_B_EvapBattTLimBexvEna) -> yTmRefriVlvCtrl_B_EvapBattTLimBexvEna/1  "yTmRefriVlvCtrl_B_EvapBattTLimBexvEna"
  Before/12(yTmRefriVlvCtrl_B_BexvCalibReq) -> yTmRefriVlvCtrl_B_BexvCalibReq/1  "yTmRefriVlvCtrl_B_BexvCalibReq"
  Before/5(sTmRefriVlvCtrl_Z_u8CEXVInitState) -> sTmRefriVlvCtrl_Z_u8CEXVInitState/1  "sTmRefriVlvCtrl_Z_u8CEXVInitState"
  Before/13(sTmRefriVlvCtrl_X_s32SM3BexvMaxPos) -> sTmRefriVlvCtrl_X_s32SM3BexvMaxPos/1  "sTmRefriVlvCtrl_X_s32SM3BexvMaxPos"
  Before/4(yTmRefriVlvCtrl_B_HpcCexvMovEnable) -> yTmRefriVlvCtrl_B_HpcCexvMovEnable/1  "yTmRefriVlvCtrl_B_HpcCexvMovEnable"
  sTmRefriVlvCtrl_D_u8EexvRefriSwitchStIn/1 -> Before/15(sTmRefriVlvCtrl_D_u8EexvRefriSwitchStIn)  "sTmRefriVlvCtrl_D_u8EexvRefriSwitchStIn"
  yTmRefriVlvCtrl_B_CexvCalibReqIn/1 -> Before/6(yTmRefriVlvCtrl_B_CexvCalibReqIn)  "yTmRefriVlvCtrl_B_CexvCalibReqIn"
  sTmRefriVlvCtrl_D_u8BexvRefriSwitchStIn/1 -> Before/17(sTmRefriVlvCtrl_D_u8BexvRefriSwitchStIn)  "sTmRefriVlvCtrl_D_u8BexvRefriSwitchStIn"
  Before/16(sTmRefriVlvCtrl_D_u8CexvRefriSwitchSt) -> Terminator/1  "sTmRefriVlvCtrl_D_u8CexvRefriSwitchSt"
  Before/2(sTmRefriVlvCtrl_X_s32EEXVPosReq) -> sTmRefriVlvCtrl_X_s32EEXVPosReq/1  "sTmRefriVlvCtrl_X_s32EEXVPosReq"
  sTmRefriVlvCtrl_D_u8CexvRefriSwitchStIn/1 -> Before/16(sTmRefriVlvCtrl_D_u8CexvRefriSwitchStIn)  "sTmRefriVlvCtrl_D_u8CexvRefriSwitchStIn"
  yTmRefriVlvCtrl_B_HpcCexvMovEnableIn/1 -> Before/4(yTmRefriVlvCtrl_B_HpcCexvMovEnableIn)  "yTmRefriVlvCtrl_B_HpcCexvMovEnableIn"
  yTmRefriVlvCtrl_B_BexvCalibReqIn/1 -> Before/12(yTmRefriVlvCtrl_B_BexvCalibReqIn)  "yTmRefriVlvCtrl_B_BexvCalibReqIn"
  Before/6(yTmRefriVlvCtrl_B_CexvCalibReq) -> yTmRefriVlvCtrl_B_CexvCalibReq/1  "yTmRefriVlvCtrl_B_CexvCalibReq"
  sTmRefriVlvCtrl_X_s32SM3BexvMaxPosIn/1 -> Before/13(sTmRefriVlvCtrl_X_s32SM3BexvMaxPosIn)  "sTmRefriVlvCtrl_X_s32SM3BexvMaxPosIn"
  yTmRefriVlvCtrl_B_HpcEexvMovEnableIn/1 -> Before/7(yTmRefriVlvCtrl_B_HpcEexvMovEnableIn)  "yTmRefriVlvCtrl_B_HpcEexvMovEnableIn"
  Ground/1 -> Before/9(yTmRefriVlvCtrl_B_EexvCalibReqIn)  "yTmRefriVlvCtrl_B_EexvCalibReqIn"
  sTmRefriVlvCtrl_Z_u8CEXVInitStateIn/1 -> Before/5(sTmRefriVlvCtrl_Z_u8CEXVInitStateIn)  "sTmRefriVlvCtrl_Z_u8CEXVInitStateIn"
  sTmRefriVlvCtrl_Z_u8BEXVInitStateIn/1 -> Before/11(sTmRefriVlvCtrl_Z_u8BEXVInitStateIn)  "sTmRefriVlvCtrl_Z_u8BEXVInitStateIn"
  sTmRefriVlvCtrl_X_s32BEXVPosReqIn/1 -> Before/3(sTmRefriVlvCtrl_X_s32BEXVPosReqIn)  "sTmRefriVlvCtrl_X_s32BEXVPosReqIn"
  Before/1(sTmRefriVlvCtrl_X_s32CEXVPosReq) -> sTmRefriVlvCtrl_X_s32CEXVPosReq/1  "sTmRefriVlvCtrl_X_s32CEXVPosReq"
  Ground1/1 -> Before/10(yTmRefriVlvCtrl_B_HpcBexvMovEnableIn)  "yTmRefriVlvCtrl_B_HpcBexvMovEnableIn"
  sTmRefriVlvCtrl_X_s32EEXVPosReqIn/1 -> Before/2(sTmRefriVlvCtrl_X_s32EEXVPosReqIn)  "sTmRefriVlvCtrl_X_s32EEXVPosReqIn"
  sTmRefriVlvCtrl_Z_u8EEXVInitStateIn/1 -> Before/8(sTmRefriVlvCtrl_Z_u8EEXVInitStateIn)  "sTmRefriVlvCtrl_Z_u8EEXVInitStateIn"
  Before/8(sTmRefriVlvCtrl_Z_u8EEXVInitState) -> sTmRefriVlvCtrl_Z_u8EEXVInitState/1  "sTmRefriVlvCtrl_Z_u8EEXVInitState"
  yTmRefriVlvCtrl_B_EvapBattTLimBexvEnaIn/1 -> Before/14(yTmRefriVlvCtrl_B_EvapBattTLimBexvEnaIn)  "yTmRefriVlvCtrl_B_EvapBattTLimBexvEnaIn"

== system ScriptDemo/Find/findNameMdOut ==
  note: [type, outName] = findNameMdOut('sTmComprCtrl_D_u32AccmKp', 'mode', 'tail')
  note: [type, outName] = findNameMdOut('sTmComprCtrl_D_u32AccmKp', 'mode', 'pre')
  SM1 : Subsystem
  SM2 : Subsystem
  SM3 : Subsystem
  SM4 : Subsystem

== system ScriptDemo/WorkFlow/Step1_CreateSoftwareReq ==
  Fun666666_Req26245_DemoSub1 : Subsystem
  Fun666666_Req26246_DemoSub2 : Subsystem
  Fun666666_Req26247_DemoSub3 : Subsystem
  Fun666666_Req26248_DemoSub4 : Subsystem
  Fun666666_Req26249_DemoSub5 : Subsystem
  Fun888888_Req26250_DemoSub6 : Subsystem
  Fun888888_Req26251_DemoSub7 : Subsystem
  Fun888888_Req26252_DemoSub8 : Subsystem
  Fun888888_Req26253_DemoSub9 : Subsystem
  Fun888888_Req26254_DemoSub10 : Subsystem
  wires:
  [sTmIn_Pw_s32HvCoolgAllwd] -> Fun666666_Req26245_DemoSub1/1(sTmIn_Pw_s32HvCoolgAllwd)
  [xTmComprCtrl_B_CompOnReqCompOn] -> Fun666666_Req26245_DemoSub1/2(xTmComprCtrl_B_CompOnReqCompOn)
  Fun666666_Req26245_DemoSub1/1(sTmComprCtrl_Pw_s32ElacCmprMaxState) -> [sTmComprCtrl_Pw_s32ElacCmprMaxState]
  Fun666666_Req26245_DemoSub1/2(yTmComprCtrl_B_HpcCoolgLimd) -> [yTmComprCtrl_B_HpcCoolgLimd]

== system ScriptDemo/WorkFlow/Step1_CreateSubModel ==
  Fun666666_Req26245_DemoSub1 : Subsystem
  Fun666666_Req26246_DemoSub2 : Subsystem
  Fun666666_Req26247_DemoSub3 : Subsystem
  Fun666666_Req26248_DemoSub4 : Subsystem
  Fun666666_Req26249_DemoSub5 : Subsystem
  Fun888888_Req26250_DemoSub6 : Subsystem
  Fun888888_Req26251_DemoSub7 : Subsystem
  Fun888888_Req26252_DemoSub8 : Subsystem
  Fun888888_Req26253_DemoSub9 : Subsystem
  Fun888888_Req26254_DemoSub10 : Subsystem

== system ScriptDemo/createHarness/After ==
  sTmDiag_D_u8CmprDischrgTFltSt : Inport  OutDataTypeStr=uint8
  sTmDiag_D_u8HiSidePFltSt : Inport  Port=2  OutDataTypeStr=uint8
  sTmDiag_D_u8OutrCondOutTFltSt : Inport  Port=3  OutDataTypeStr=uint8
  sTmIn_D_u8HeatPump : Inport  Port=4  OutDataTypeStr=uint8
  sTmDiag_D_u8HiSidePNHPFltSt : Inport  Port=5  OutDataTypeStr=uint8
  Compare To Constant : simulink/Logic and Bit Operations/Compare To Constant  relop=~=  const=0  OutDataTypeStr=boolean
  Compare To Constant1 : simulink/Logic and Bit Operations/Compare To Constant  relop=~=  const=0  OutDataTypeStr=boolean
  Compare To Constant2 : simulink/Logic and Bit Operations/Compare To Constant  relop=~=  const=0  OutDataTypeStr=boolean
  Compare To Constant3 : simulink/Logic and Bit Operations/Compare To Constant  relop===  const=2  OutDataTypeStr=boolean
  Compare To Constant4 : simulink/Logic and Bit Operations/Compare To Constant  relop===  const=2  OutDataTypeStr=boolean
  Compare To Constant5 : simulink/Logic and Bit Operations/Compare To Constant  relop===  const=2  OutDataTypeStr=boolean
  Compare To Constant6 : simulink/Logic and Bit Operations/Compare To Constant  relop===  const=[1 2 3]  OutDataTypeStr=boolean
  Compare To Constant7 : simulink/Logic and Bit Operations/Compare To Constant  relop===  const=1  OutDataTypeStr=boolean
  Constant : Constant  Value=cTmComprCtrl_n_u16CmpMaxSpdSensorFltLimt  OutDataTypeStr=uint16
  Constant1 : Constant  Value=8000  OutDataTypeStr=uint16
  Logical Operator : Logic  Operator=OR  Inputs=4  AllPortsSameDT=off  OutDataTypeStr=boolean
  Logical Operator{1..4} (4 alike) : Logic  AllPortsSameDT=off  OutDataTypeStr=boolean
  Logical Operator5 : Logic  Operator=OR  Inputs=1  AllPortsSameDT=off  OutDataTypeStr=boolean
  Switch : Switch  Criteria=u2 ~= 0  SaturateOnIntegerOverflow=off  InputSameDT=off
  rTmComprCtrl_n_u16CompMaxRpmSensFlt : Outport  OutDataTypeStr=uint16
  xTmComprCtrl_B_CmpSensorFltLimtFlag : Outport  Port=2  OutDataTypeStr=boolean
  wires:
  [sTmDiag_D_u8HiSidePFltSt] -> Compare To Constant/1
  [sTmDiag_D_u8OutrCondOutTFltSt] -> Compare To Constant1/1
  [sTmDiag_D_u8CmprDischrgTFltSt] -> Compare To Constant2/1
  Constant/1 -> Switch/1
  Switch/1 -> [rTmComprCtrl_n_u16CompMaxRpmSensFlt]  "rTmComprCtrl_n_u16CompMaxRpmSensFlt"
  Constant1/1 -> Switch/3
  sTmDiag_D_u8CmprDischrgTFltSt/1 -> [sTmDiag_D_u8CmprDischrgTFltSt]  "sTmDiag_D_u8CmprDischrgTFltSt"
  sTmDiag_D_u8HiSidePFltSt/1 -> [sTmDiag_D_u8HiSidePFltSt]  "sTmDiag_D_u8HiSidePFltSt"
  sTmDiag_D_u8OutrCondOutTFltSt/1 -> [sTmDiag_D_u8OutrCondOutTFltSt]  "sTmDiag_D_u8OutrCondOutTFltSt"
  [rTmComprCtrl_n_u16CompMaxRpmSensFlt] -> rTmComprCtrl_n_u16CompMaxRpmSensFlt/1  "rTmComprCtrl_n_u16CompMaxRpmSensFlt"
  Logical Operator/1 -> [xTmComprCtrl_B_CmpSensorFltLimtFlag]
  [xTmComprCtrl_B_CmpSensorFltLimtFlag] -> xTmComprCtrl_B_CmpSensorFltLimtFlag/1  "xTmComprCtrl_B_CmpSensorFltLimtFlag"
  [xTmComprCtrl_B_CmpSensorFltLimtFlag] -> Switch/2
  [sTmIn_D_u8HeatPump] -> Compare To Constant3/1
  Compare To Constant3/1 -> Logical Operator1/1
  Compare To Constant1/1 -> Logical Operator1/2
  [sTmIn_D_u8HeatPump] -> Compare To Constant4/1
  Compare To Constant4/1 -> Logical Operator2/1
  Compare To Constant2/1 -> Logical Operator2/2
  sTmIn_D_u8HeatPump/1 -> [sTmIn_D_u8HeatPump]  "sTmIn_D_u8HeatPump"
  [sTmIn_D_u8HeatPump] -> Compare To Constant5/1
  Compare To Constant/1 -> Logical Operator3/2
  Compare To Constant5/1 -> Logical Operator3/1
  Compare To Constant6/1 -> Logical Operator5/1
  [sTmIn_D_u8HeatPump] -> Compare To Constant7/1
  [sTmDiag_D_u8HiSidePNHPFltSt] -> Compare To Constant6/1
  Compare To Constant7/1 -> Logical Operator4/1
  Logical Operator1/1 -> Logical Operator/3
  Logical Operator2/1 -> Logical Operator/4
  Logical Operator3/1 -> Logical Operator/2
  Logical Operator4/1 -> Logical Operator/1
  sTmDiag_D_u8HiSidePNHPFltSt/1 -> [sTmDiag_D_u8HiSidePNHPFltSt]  "sTmDiag_D_u8HiSidePNHPFltSt"
  Logical Operator5/1 -> Logical Operator4/2

== system ScriptDemo/createHarness/Before ==
  sTmDiag_D_u8CmprDischrgTFltSt : Inport  OutDataTypeStr=uint8
  sTmDiag_D_u8HiSidePFltSt : Inport  Port=2  OutDataTypeStr=uint8
  sTmDiag_D_u8OutrCondOutTFltSt : Inport  Port=3  OutDataTypeStr=uint8
  sTmIn_D_u8HeatPump : Inport  Port=4  OutDataTypeStr=uint8
  sTmDiag_D_u8HiSidePNHPFltSt : Inport  Port=5  OutDataTypeStr=uint8
  Compare To Constant : simulink/Logic and Bit Operations/Compare To Constant  relop=~=  const=0  OutDataTypeStr=boolean
  Compare To Constant1 : simulink/Logic and Bit Operations/Compare To Constant  relop=~=  const=0  OutDataTypeStr=boolean
  Compare To Constant2 : simulink/Logic and Bit Operations/Compare To Constant  relop=~=  const=0  OutDataTypeStr=boolean
  Compare To Constant3 : simulink/Logic and Bit Operations/Compare To Constant  relop===  const=2  OutDataTypeStr=boolean
  Compare To Constant4 : simulink/Logic and Bit Operations/Compare To Constant  relop===  const=2  OutDataTypeStr=boolean
  Compare To Constant5 : simulink/Logic and Bit Operations/Compare To Constant  relop===  const=2  OutDataTypeStr=boolean
  Compare To Constant6 : simulink/Logic and Bit Operations/Compare To Constant  relop===  const=[1 2 3]  OutDataTypeStr=boolean
  Compare To Constant7 : simulink/Logic and Bit Operations/Compare To Constant  relop===  const=1  OutDataTypeStr=boolean
  Constant : Constant  Value=cTmComprCtrl_n_u16CmpMaxSpdSensorFltLimt  OutDataTypeStr=uint16
  Constant1 : Constant  Value=8000  OutDataTypeStr=uint16
  Logical Operator : Logic  Operator=OR  Inputs=4  AllPortsSameDT=off  OutDataTypeStr=boolean
  Logical Operator{1..4} (4 alike) : Logic  AllPortsSameDT=off  OutDataTypeStr=boolean
  Switch : Switch  Criteria=u2 ~= 0  SaturateOnIntegerOverflow=off  InputSameDT=off
  rTmComprCtrl_n_u16CompMaxRpmSensFlt : Outport  OutDataTypeStr=uint16
  xTmComprCtrl_B_CmpSensorFltLimtFlag : Outport  Port=2  OutDataTypeStr=boolean
  wires:
  [sTmDiag_D_u8HiSidePFltSt] -> Compare To Constant/1
  [sTmDiag_D_u8OutrCondOutTFltSt] -> Compare To Constant1/1
  [sTmDiag_D_u8CmprDischrgTFltSt] -> Compare To Constant2/1
  Constant/1 -> Switch/1
  Switch/1 -> [rTmComprCtrl_n_u16CompMaxRpmSensFlt]  "rTmComprCtrl_n_u16CompMaxRpmSensFlt"
  Constant1/1 -> Switch/3
  sTmDiag_D_u8CmprDischrgTFltSt/1 -> [sTmDiag_D_u8CmprDischrgTFltSt]  "sTmDiag_D_u8CmprDischrgTFltSt"
  sTmDiag_D_u8HiSidePFltSt/1 -> [sTmDiag_D_u8HiSidePFltSt]  "sTmDiag_D_u8HiSidePFltSt"
  sTmDiag_D_u8OutrCondOutTFltSt/1 -> [sTmDiag_D_u8OutrCondOutTFltSt]  "sTmDiag_D_u8OutrCondOutTFltSt"
  [rTmComprCtrl_n_u16CompMaxRpmSensFlt] -> rTmComprCtrl_n_u16CompMaxRpmSensFlt/1  "rTmComprCtrl_n_u16CompMaxRpmSensFlt"
  Logical Operator/1 -> [xTmComprCtrl_B_CmpSensorFltLimtFlag]
  [xTmComprCtrl_B_CmpSensorFltLimtFlag] -> xTmComprCtrl_B_CmpSensorFltLimtFlag/1  "xTmComprCtrl_B_CmpSensorFltLimtFlag"
  [xTmComprCtrl_B_CmpSensorFltLimtFlag] -> Switch/2
  [sTmIn_D_u8HeatPump] -> Compare To Constant3/1
  Compare To Constant3/1 -> Logical Operator1/1
  Compare To Constant1/1 -> Logical Operator1/2
  [sTmIn_D_u8HeatPump] -> Compare To Constant4/1
  Compare To Constant4/1 -> Logical Operator2/1
  Compare To Constant2/1 -> Logical Operator2/2
  sTmIn_D_u8HeatPump/1 -> [sTmIn_D_u8HeatPump]  "sTmIn_D_u8HeatPump"
  [sTmIn_D_u8HeatPump] -> Compare To Constant5/1
  Compare To Constant/1 -> Logical Operator3/2
  Compare To Constant5/1 -> Logical Operator3/1
  Compare To Constant6/1 -> Logical Operator4/2
  [sTmIn_D_u8HeatPump] -> Compare To Constant7/1
  [sTmDiag_D_u8HiSidePNHPFltSt] -> Compare To Constant6/1
  Compare To Constant7/1 -> Logical Operator4/1
  Logical Operator1/1 -> Logical Operator/3
  Logical Operator2/1 -> Logical Operator/4
  Logical Operator3/1 -> Logical Operator/2
  Logical Operator4/1 -> Logical Operator/1
  sTmDiag_D_u8HiSidePNHPFltSt/1 -> [sTmDiag_D_u8HiSidePNHPFltSt]  "sTmDiag_D_u8HiSidePNHPFltSt"

== system ScriptDemo/createHarness/Blue ==
  sTmDiag_D_u8CmprDischrgTFltSt : Inport  OutDataTypeStr=uint8
  sTmDiag_D_u8HiSidePFltSt : Inport  Port=2  OutDataTypeStr=uint8
  sTmDiag_D_u8OutrCondOutTFltSt : Inport  Port=3  OutDataTypeStr=uint8
  sTmIn_D_u8HeatPump : Inport  Port=4  OutDataTypeStr=uint8
  sTmDiag_D_u8HiSidePNHPFltSt : Inport  Port=5  OutDataTypeStr=uint8
  Compare To Constant : simulink/Logic and Bit Operations/Compare To Constant  relop=~=  const=0  OutDataTypeStr=boolean
  Compare To Constant1 : simulink/Logic and Bit Operations/Compare To Constant  relop=~=  const=0  OutDataTypeStr=boolean
  Compare To Constant2 : simulink/Logic and Bit Operations/Compare To Constant  relop=~=  const=0  OutDataTypeStr=boolean
  Compare To Constant3 : simulink/Logic and Bit Operations/Compare To Constant  relop===  const=2  OutDataTypeStr=boolean
  Compare To Constant4 : simulink/Logic and Bit Operations/Compare To Constant  relop===  const=2  OutDataTypeStr=boolean
  Compare To Constant5 : simulink/Logic and Bit Operations/Compare To Constant  relop===  const=2  OutDataTypeStr=boolean
  Compare To Constant6 : simulink/Logic and Bit Operations/Compare To Constant  relop===  const=[1 2 3]  OutDataTypeStr=boolean
  Compare To Constant7 : simulink/Logic and Bit Operations/Compare To Constant  relop===  const=1  OutDataTypeStr=boolean
  Constant : Constant  Value=cTmComprCtrl_n_u16CmpMaxSpdSensorFltLimt  OutDataTypeStr=uint16
  Constant1 : Constant  Value=8000  OutDataTypeStr=uint16
  Logical Operator : Logic  Operator=OR  Inputs=4  AllPortsSameDT=off  OutDataTypeStr=boolean
  Logical Operator{1..4} (4 alike) : Logic  AllPortsSameDT=off  OutDataTypeStr=boolean
  Logical Operator5 : Logic  Operator=OR  Inputs=1  AllPortsSameDT=off  OutDataTypeStr=boolean
  Switch : Switch  Criteria=u2 ~= 0  SaturateOnIntegerOverflow=off  InputSameDT=off
  rTmComprCtrl_n_u16CompMaxRpmSensFlt : Outport  OutDataTypeStr=uint16
  xTmComprCtrl_B_CmpSensorFltLimtFlag : Outport  Port=2  OutDataTypeStr=boolean
  wires:
  [sTmDiag_D_u8HiSidePFltSt] -> Compare To Constant/1
  [sTmDiag_D_u8OutrCondOutTFltSt] -> Compare To Constant1/1
  [sTmDiag_D_u8CmprDischrgTFltSt] -> Compare To Constant2/1
  Constant/1 -> Switch/1
  Switch/1 -> [rTmComprCtrl_n_u16CompMaxRpmSensFlt]  "rTmComprCtrl_n_u16CompMaxRpmSensFlt"
  Constant1/1 -> Switch/3
  sTmDiag_D_u8CmprDischrgTFltSt/1 -> [sTmDiag_D_u8CmprDischrgTFltSt]
  sTmDiag_D_u8HiSidePFltSt/1 -> [sTmDiag_D_u8HiSidePFltSt]
  sTmDiag_D_u8OutrCondOutTFltSt/1 -> [sTmDiag_D_u8OutrCondOutTFltSt]
  [rTmComprCtrl_n_u16CompMaxRpmSensFlt] -> rTmComprCtrl_n_u16CompMaxRpmSensFlt/1
  Logical Operator/1 -> [xTmComprCtrl_B_CmpSensorFltLimtFlag]
  [xTmComprCtrl_B_CmpSensorFltLimtFlag] -> xTmComprCtrl_B_CmpSensorFltLimtFlag/1
  [xTmComprCtrl_B_CmpSensorFltLimtFlag] -> Switch/2
  [sTmIn_D_u8HeatPump] -> Compare To Constant3/1
  Compare To Constant3/1 -> Logical Operator1/1
  Compare To Constant1/1 -> Logical Operator1/2
  [sTmIn_D_u8HeatPump] -> Compare To Constant4/1
  Compare To Constant4/1 -> Logical Operator2/1
  Compare To Constant2/1 -> Logical Operator2/2
  sTmIn_D_u8HeatPump/1 -> [sTmIn_D_u8HeatPump]
  [sTmIn_D_u8HeatPump] -> Compare To Constant5/1
  Compare To Constant/1 -> Logical Operator3/2
  Compare To Constant5/1 -> Logical Operator3/1
  Compare To Constant6/1 -> Logical Operator5/1
  [sTmIn_D_u8HeatPump] -> Compare To Constant7/1
  [sTmDiag_D_u8HiSidePNHPFltSt] -> Compare To Constant6/1
  Compare To Constant7/1 -> Logical Operator4/1
  Logical Operator1/1 -> Logical Operator/3
  Logical Operator2/1 -> Logical Operator/4
  Logical Operator3/1 -> Logical Operator/2
  Logical Operator4/1 -> Logical Operator/1
  sTmDiag_D_u8HiSidePNHPFltSt/1 -> [sTmDiag_D_u8HiSidePNHPFltSt]
  Logical Operator5/1 -> Logical Operator4/2

== system ScriptDemo/createHarness/ID31659_OffCodeState ==
  sTmComprCtrl_D_u32AcOffCode : Inport  OutDataTypeStr=uint32
  sTmComprCtrl_D_u32AcOffCode2 : Inport  Port=2  OutDataTypeStr=uint32
  Bias : Bias  Bias=32  SaturateOnIntegerOverflow=off
  Compare To Constant : simulink/Logic and Bit Operations/Compare To Constant  relop=~=  const=0  OutDataTypeStr=boolean
  Compare To Constant1 : simulink/Logic and Bit Operations/Compare To Constant  relop===  const=0  OutDataTypeStr=boolean
  Data Type Conversion : DataTypeConversion  OutDataTypeStr=uint8  SaturateOnIntegerOverflow=off  RndMeth=Floor
  Data Type Conversion1 : DataTypeConversion  OutDataTypeStr=uint8  SaturateOnIntegerOverflow=off  RndMeth=Floor
  Logical Operator : Logic  Operator=OR  AllPortsSameDT=off  OutDataTypeStr=boolean
  MATLAB Function : MATLAB Function  TreatAsAtomicUnit=on
  MATLAB Function1 : MATLAB Function  TreatAsAtomicUnit=on
  MATLAB Function2 : MATLAB Function  Commented=on  TreatAsAtomicUnit=on
  Switch : Switch  Criteria=u2 ~= 0  SaturateOnIntegerOverflow=off  InputSameDT=off
  Switch1 : Switch  Criteria=u2 ~= 0  SaturateOnIntegerOverflow=off  InputSameDT=off
  Unit Delay : UnitDelay  SampleTime=-1  HasFrameUpgradeWarning=on
  bk : Subsystem  Commented=on
  sTmComprCtrl_D_u8ACOffState : Outport  OutDataTypeStr=uint8
  wires:
  sTmComprCtrl_D_u32AcOffCode/1 -> Compare To Constant/1, MATLAB Function/1(num)  "sTmComprCtrl_D_u32AcOffCode"
  MATLAB Function/1(pos) -> Data Type Conversion/1
  sTmComprCtrl_D_u32AcOffCode2/1 -> Compare To Constant1/1, MATLAB Function1/1(num)  "sTmComprCtrl_D_u32AcOffCode2"
  MATLAB Function1/1(pos) -> Data Type Conversion1/1
  Data Type Conversion/1 -> Switch/1
  Data Type Conversion1/1 -> Bias/1
  Bias/1 -> Switch/3
  Compare To Constant/1 -> Logical Operator/1
  Compare To Constant1/1 -> Logical Operator/2
  Logical Operator/1 -> Switch/2
  Switch/1 -> Switch1/1, Switch1/2
  Switch1/1 -> sTmComprCtrl_D_u8ACOffState/1, Unit Delay/1  "sTmComprCtrl_D_u8ACOffState"
  Unit Delay/1 -> Switch1/3

== system ScriptDemo/Change/changeModPortName/After ==
  sTmSigProces_Te_s32EvapFanReqRamp : Inport  OutDataTypeStr=single
  sTmDiag_D_u8TeEvapFltSt : Inport  Port=2  OutDataTypeStr=uint8
  sTmIn_D_u8HeatPump : Inport  Port=3  OutDataTypeStr=uint8
  sTmIn_X_s32ClimtRcirc : Inport  Port=4  OutDataTypeStr=single
  sTmComprCtrl_D_u8HvacFlowLevel : Inport  Port=5  OutDataTypeStr=uint8
  sTmSigProces_Te_s32EvapFanFilter : Inport  Port=6  OutDataTypeStr=single
  sTmSigProces_Te_s32SatLp : Inport  Port=7  OutDataTypeStr=single
  xTmComprCtrl_B_CompOnReqCompOn : Inport  Port=8  OutDataTypeStr=boolean
  yTmRefriModeMgr_B_CoolOCRMode : Inport  Port=9  OutDataTypeStr=boolean
  sTmSigProces_Pw_i16ReqPwrForCool : Inport  Port=10  OutDataTypeStr=int16
  rSM2SM22_n_u16DisOverrideValue : Outport  OutDataTypeStr=uint16
  rSM2SM22_t_u16PIPeriod : Outport  Port=2  OutDataTypeStr=uint16
  rSM2SM22_Te_s32UpErrStop : Outport  Port=3  OutDataTypeStr=single
  rSM2SM22_n_u16ComprRpmFF : Outport  Port=4  OutDataTypeStr=uint16
  rSM2SM22_n_u16ComprRpmKp : Outport  Port=5  OutDataTypeStr=uint16
  rSM2SM22_n_u16ComprRpmKi : Outport  Port=6  OutDataTypeStr=uint16
  rSM2SM22_Te_s32LowErrStop : Outport  Port=7  OutDataTypeStr=single
  rSM2SM22_n_i16KpUpLimit : Outport  Port=8  OutDataTypeStr=int16
  rSM2SM22_n_i16KpLowLimit : Outport  Port=9  OutDataTypeStr=int16
  rSM2SM22_n_i16KiUpLimit : Outport  Port=10  OutDataTypeStr=int16
  rSM2SM22_n_i16KiLowLimit : Outport  Port=11  OutDataTypeStr=int16
  rSM2SM22_B_Enable : Outport  Port=12  OutDataTypeStr=boolean
  rSM2SM22_Te_s32TempError : Outport  Port=13  OutDataTypeStr=single
  wires:
  sTmSigProces_Te_s32EvapFanReqRamp/1 -> [sTmSigProces_Te_s32EvapFanReqRamp]
  sTmDiag_D_u8TeEvapFltSt/1 -> [sTmDiag_D_u8TeEvapFltSt]
  sTmIn_D_u8HeatPump/1 -> [sTmIn_D_u8HeatPump]
  ? -> [sTmSigProces_Te_s32TAmb]
  sTmIn_X_s32ClimtRcirc/1 -> [sTmIn_X_s32ClimtRcirc]
  sTmComprCtrl_D_u8HvacFlowLevel/1 -> [sTmComprCtrl_D_u8HvacFlowLevel]
  sTmSigProces_Te_s32EvapFanFilter/1 -> [sTmSigProces_Te_s32EvapFanFilter]
  sTmSigProces_Te_s32SatLp/1 -> [sTmSigProces_Te_s32SatLp]
  xTmComprCtrl_B_CompOnReqCompOn/1 -> [xTmComprCtrl_B_CompOnReqCompOn]
  ? -> [yTmRefriModeMgr_B_CoolModeInCycle]
  [rTmComprCtrl_n_u16DisOverrideValue] -> rSM2SM22_n_u16DisOverrideValue/1
  [rTmComprCtrl_t_u16PIPeriod] -> rSM2SM22_t_u16PIPeriod/1
  [rTmComprCtrl_Te_s32UpErrStop] -> rSM2SM22_Te_s32UpErrStop/1
  [rTmComprCtrl_n_u16ComprRpmFF] -> rSM2SM22_n_u16ComprRpmFF/1
  [rTmComprCtrl_n_u16ComprRpmKp] -> rSM2SM22_n_u16ComprRpmKp/1
  [rTmComprCtrl_n_u16ComprRpmKi] -> rSM2SM22_n_u16ComprRpmKi/1
  [rTmComprCtrl_Te_s32LowErrStop] -> rSM2SM22_Te_s32LowErrStop/1
  [rTmComprCtrl_n_i16KpUpLimit] -> rSM2SM22_n_i16KpUpLimit/1
  [rTmComprCtrl_n_i16KpLowLimit] -> rSM2SM22_n_i16KpLowLimit/1
  [rTmComprCtrl_n_i16KiUpLimit] -> rSM2SM22_n_i16KiUpLimit/1
  [rTmComprCtrl_n_i16KiLowLimit] -> rSM2SM22_n_i16KiLowLimit/1
  [xTmComprCtrl_B_Enable] -> rSM2SM22_B_Enable/1
  [rTmComprCtrl_Te_s32TempError] -> rSM2SM22_Te_s32TempError/1
  yTmRefriModeMgr_B_CoolOCRMode/1 -> [yTmRefriModeMgr_B_CoolOCRMode]
  sTmSigProces_Pw_i16ReqPwrForCool/1 -> [sTmSigProces_Pw_i16ReqPwrForCool]
